simulink model "PassengerCar"  (R2019b)
settings: Solver=ode1  StartTime=0  StopTime=25  FixedStep=1.0000000000000000e-003  RelTol=1e-3
InitFcn:
  | sampleTime = str2double(get_param(bdroot, 'FixedStep'));
undefined symbols (not defined in the file or in its folder): AccPedalPos, BrakePedalPos, BrakeSwitch, DiscIntNeverNeededParam, DYNA4, EngSpd, IgnitionSwitch, InitialGear, InitialSpeed, IntendedEngTrq, LeftIndicator, MainBrakePress, MaxGear, MDL, MinGear, RefAcc, RefLane, RefLatPos, RefPath, RefPathCurv, RefSpd, RefSpdPreview, RefSpdRetrospect, RightIndicator, SteeringWheelAng, SteeringWheelTrq, UserDefinedRefValue, vm_const
libraries: UtilitiesLibrary x31, simulink x18, WheelSystemModules x13, LongitudinalControllerModules x13, LateralControllerModules x7, AnimationBusselectorModules x5, EnvironmentModules x5, BasicEngineControlModules x5, MiscellaneousControlModules x5, Animation3Modules x4, AuxiliariesModules x4, TireModules x4
(part 2 of 39)

== system PassengerCar/Animation ==
  fromCTRL : Inport
  fromControlUnits : Inport  Port=2
  fromTrailer : Inport  Port=3
  fromVehicle : Inport  Port=4
  fromTraffic : Inport  Port=5
  Animation3 : Animation3Modules/Animation3  DATA_NODE=MDL.Animation.Animation3
  AnimationContent : Animation3Modules/AnimationContentGeneric  SystemSampleTime=-1  Latency=0  AutoFrameSizeCalculation=off
  Bus Creator : BusCreator  Inputs=4
  DynaComponentInfo : Subsystem  Tag=DynaComponentInfo
      mask init:
      | data= get_param(gcb, 'UserData');
      settings: OpenFcn=DYNA4.ModelHandling.Component.ShowEditComponentInformationDialog(gcb);
      mask Display: disp(['Type = ', data.type, '\nGroup = ', data.group, '\nName = ', data.name ])
  Gauge Signals : AnimationBusselectorModules/Gauge Signals  SystemSampleTime=-1  Latency=0  AutoFrameSizeCalculation=off
  Open AnimationBusselectorModules : AnimationBusselectorModules/Open AnimationBusselectorModules  SystemSampleTime=-1  Latency=0  AutoFrameSizeCalculation=off
  Scenario Design : AnimationBusselectorModules/Scenario Design  SystemSampleTime=-1  Latency=0  AutoFrameSizeCalculation=off
  Terminator : Terminator
  Terminator1 : Terminator
  Terminator2 : Terminator
  Vehicle Light Signals : AnimationBusselectorModules/Vehicle Light Signals  SystemSampleTime=-1  VariantControl=AnimationData_Lights  Latency=0  AutoFrameSizeCalculation=off
  Vehicle Signals With Axles Animation : AnimationBusselectorModules/Vehicle Signals With Axles Animation  SystemSampleTime=-1  Latency=0  AutoFrameSizeCalculation=off
      settings: AttributesFormatString=requires veDYNA Chassis Component signals!
  wires:
  fromVehicle/1 -> Scenario Design/1, Vehicle Signals With Axles Animation/1, Gauge Signals/1
  fromCTRL/1 -> Scenario Design/2, Vehicle Light Signals/1
  fromTrailer/1 -> Terminator1/1
  fromControlUnits/1 -> Terminator2/1
  Vehicle Light Signals/1 -> Bus Creator/3
  Vehicle Signals With Axles Animation/1 -> Bus Creator/2
  Gauge Signals/1 -> Bus Creator/1
  Bus Creator/1 -> Animation3/1
  fromTraffic/1 -> Terminator/1
  Scenario Design/1 -> Bus Creator/4

== system PassengerCar/ComponentsOutput ==
  ControlUnits___UNIQUE_1 : Inport  Description=|
      | <name>ControlUnits</name>
      | <comment></comment>
  Trailer___UNIQUE_1 : Inport  Description=|  Port=2
      | <name>Trailer</name>
      | <comment></comment>
  Vehicle___UNIQUE_1 : Inport  Description=|  Port=3
      | <name>Vehicle</name>
      | <comment></comment>
  Environment___UNIQUE_1 : Inport  Description=|  Port=4
      | <name>Environment</name>
      | <comment></comment>
  Traffic___UNIQUE_1 : Inport  Description=|  Port=5
      | <name>Traffic</name>
      | <comment></comment>
  VehicleControl___UNIQUE_1 : Inport  Description=|  Port=6
      | <name>VehicleControl</name>
      | <comment></comment>
  __SRC__Components.(none) : Constant  Value=0.0  OutDataTypeStr=Inherit: Inherit via back propagation
  __TDO__Components : BusCreator  Inputs=7
  Components___UNIQUE_1 : Outport  Tag=TESIS DYNAware Component Bus Root  Description=|  VectorParamsAs1DForOutWhenUnconnected=off
      | <name></name>
      | <comment></comment>
  wires:
  __SRC__Components.(none)/1 -> __TDO__Components/1  "(none)"
  ControlUnits___UNIQUE_1/1 -> __TDO__Components/2  "ControlUnits"
  Trailer___UNIQUE_1/1 -> __TDO__Components/3  "Trailer"
  Vehicle___UNIQUE_1/1 -> __TDO__Components/4  "Vehicle"
  Environment___UNIQUE_1/1 -> __TDO__Components/5  "Environment"
  Traffic___UNIQUE_1/1 -> __TDO__Components/6  "Traffic"
  VehicleControl___UNIQUE_1/1 -> __TDO__Components/7  "VehicleControl"
  __TDO__Components/1 -> Components___UNIQUE_1/1  "Components"

== system PassengerCar/ControlUnits ==
  note: This component contains central control units that usually use bus communication
      | in the real vehicle to communicate with their physical counterpart.
      | Control units that are directly connected to their hardware counterpart such as
      | BrakeSystemControlUnit are located next to the corresponding physical component.
  fromCTRL : Inport
  fromTrailer : Inport  Port=2
  fromVehicle : Inport  Port=3
  fromTraffic : Inport  Port=4
  ADAS : Subsystem
  ControlUnitsOutput : Subsystem  Tag=TESIS DYNAware Interface Block  mask{NeedsUpdate=off, SignalInfo=|}
      mask SignalInfo=|
      | {
      |   "Version": "4.6",
      |   "MuxedOutputBusName": "ControlUnits",
      |   "MuxedInputBusName": "input",
      |   "MuxedInputSelected": false,
      |   "MuxedOutputSelected": true,
      |   "SignalData": [
      |     {
      |       "initialValue": "0.0",
      |       "name": "VCU",
      |       "comment": "",
      |       "minString": "",
      |       "maxString": "",
      |       "width": -1,
      |       "dataType": 0,
      |       "signalType": 1,
      |       "createSignal": false,
      |       "outputName": "VCU",
      |       "generateSignalAccessBlock": false,
      |       "accessId": "$(parentId).$(blockName).$(outputName)"
      |     },
      |     {
      |       "initialValue": "0.0",
      |       "name": "ADAS",
      |       "comment": "",
      |       "minString": "",
      |       "maxString": "",
      |       "width": -1,
      |       "dataType": 0,
      |       "signalType": 1,
      |       "createSignal": false,
      |       "outputName": "ADAS",
      |       "generateSignalAccessBlock": false,
      |       "accessId": "$(parentId).$(blockName).$(outputName)"
      |     },
      |     {
      |       "initialValue": "0.0",
      |       "name": "LCU",
      |       "comment": "",
      |       "minString": "",
      |       "maxString": "",
      |       "width": -1,
      |       "dataType": 0,
      |       "signalType": 1,
      |       "createSignal": false,
      |       "outputName": "LCU",
      |       "generateSignalAccessBlock": false,
      |       "accessId": "$(parentId).$(blockName).$(outputName)"
      |     },
      |     {
      |       "initialValue": "0.0",
      |       "name": "StateSensors",
      |       "comment": "",
      |       "minString": "",
      |       "maxString": "",
      |       "width": -1,
      |       "dataType": 0,
      |       "signalType": 1,
      |       "createSignal": false,
      |       "outputName": "StateSensors",
      |       "generateSignalAccessBlock": false,
      |       "accessId": "$(parentId).$(blockName).$(outputName)"
      |     }
      |   ]
      | }
      mask prompts: NeedsUpdate "Specify, if subsystem content needs to be updated"; SignalInfo "Signal Info (json)"
      mask help: DYNA4 Interface Block Version 4.6
      mask init:
      | blockName = get_param(gcbh, 'Name');
      | parentId = DYNA4.ModelHandling.AccessID.getFromHierarchy(gcbh);
      | TD.InterfaceBlock.ModelCallbacks.GenerateContent(gcb);
      settings: DeleteFcn=TD.InterfaceBlock.ModelCallbacks.CloseGUI( gcbh );  NameChangeFcn=TD.InterfaceBlock.ModelCallbacks.BlockRenamedHandler(gcbh);  OpenFcn=TD.InterfaceBlock.ModelCallbacks.OpenGUI( gcbh );  CloseFcn=TD.InterfaceBlock.ModelCallbacks.CloseGUI( gcbh );
      mask Display:
      | image('InterfaceBlock.png','center');
      | port_label('input',1, 'VCU');
      | port_label('input',2, 'ADAS');
      | port_label('input',3, 'LCU');
      | port_label('input',4, 'StateSensors');
      | port_label('output',1, 'ControlUnits');
  DynaComponentInfo : Subsystem  Tag=DynaComponentInfo
      mask init:
      | data= get_param(gcb, 'UserData');
      settings: OpenFcn=DYNA4.ModelHandling.Component.ShowEditComponentInformationDialog(gcb);
      mask Display: disp(['Type = ', data.type, '\nGroup = ', data.group, '\nName = ', data.name ])
  LCU : Subsystem
  StateSensors : Subsystem
  TraceMarker : UtilitiesLibrary/DYNA4 Trace Marker  Tag=DYNA4_TRACE_MARKER  SettingType=Standard  PrefixModelBlockID=on  PrefixRootSignalName=off  NamePattern='$(modelBlockID).$(rootSignalName)'
  VCU : Subsystem
  ControlUnits : Outport  VectorParamsAs1DForOutWhenUnconnected=off
  wires:
  fromTraffic/1 -> StateSensors/4(fromTraffic)
  fromTrailer/1 -> StateSensors/2(fromTrailer)
  fromVehicle/1 -> ADAS/2(fromVehicle), LCU/2(fromVehicle), StateSensors/3(fromVehicle), VCU/2(fromVehicle)
  fromCTRL/1 -> ADAS/1(fromCTRL), LCU/1(fromCTRL), StateSensors/1(fromCTRL), VCU/1(fromCTRL)
  LCU/1(LCU) -> ControlUnitsOutput/3(LCU___UNIQUE_1)
  ControlUnitsOutput/1(ControlUnits___UNIQUE_1) -> ControlUnits/1, TraceMarker/1
  ADAS/1(ADAS) -> ControlUnitsOutput/2(ADAS___UNIQUE_1), VCU/3(fromADAS)
  VCU/1(VCU) -> ControlUnitsOutput/1(VCU___UNIQUE_1)
  StateSensors/1(StateSensors) -> ControlUnitsOutput/4(StateSensors___UNIQUE_1)

== system PassengerCar/DYNA4 Logo ==

== system PassengerCar/Environment ==
  fromCTRL : Inport
  fromTrailer : Inport  Port=2
  fromVehicle : Inport  Port=3
  fromTraffic : Inport  Port=4
  AdditionalRoadElevation : EnvironmentModules/AdditionalRoadElevation  DATA_NODE=MDL.Environment.AdditionalRoadElevation  AddLongRoadSlope=MDL.Environment.AdditionalRoadElevation.AddLongRoadSlope  AddLatRoadSlope=MDL.Environment.AdditionalRoadElevation.AddLatRoadSlope  FrontLeftAddRoadElev=MDL.Environment.AdditionalRoadElevation.FrontLeftAddRoadElev  FrontRightAddRoadElev=MDL.Environment.AdditionalRoadElevation.FrontRightAddRoadElev  RearLeftAddRoadElev=MDL.Environment.AdditionalRoadElevation.RearLeftAddRoadElev  RearRightAddRoadElev=MDL.Environment.AdditionalRoadElevation.RearRightAddRoadElev  Rear2LeftAddRoadElev=MDL.Environment.AdditionalRoadElevation.Rear2LeftAddRoadElev  Rear2RightAddRoadElev=MDL.Environment.AdditionalRoadElevation.Rear2RightAddRoadElev  Rear3LeftAddRoadElev=MDL.Environment.AdditionalRoadElevation.Rear3LeftAddRoadElev  Rear3RightAddRoadElev=MDL.Environment.AdditionalRoadElevation.Rear3RightAddRoadElev  TrailerFrontLeftAddRoadElev=MDL.Environment.AdditionalRoadElevation.TrailerFrontLeftAddRoadElev  TrailerFrontRightAddRoadElev=MDL.Environment.AdditionalRoadElevation.TrailerFrontRightAddRoadElev  TrailerRearLeftAddRoadElev=MDL.Environment.AdditionalRoadElevation.TrailerRearLeftAddRoadElev  TrailerRearRightAddRoadElev=MDL.Environment.AdditionalRoadElevation.TrailerRearRightAddRoadElev  TrailerRear2LeftAddRoadElev=MDL.Environment.AdditionalRoadElevation.TrailerRear2LeftAddRoadElev  TrailerRear2RightAddRoadElev=MDL.Environment.AdditionalRoadElevation.TrailerRear2RightAddRoadElev  TrailerRear3LeftAddRoadElev=MDL.Environment.AdditionalRoadElevation.TrailerRear3LeftAddRoadElev  TrailerRear3RightAddRoadElev=MDL.Environment.AdditionalRoadElevation.TrailerRear3RightAddRoadElev  AbscissaTypes=MDL.Environment.AdditionalRoadElevation.AbscissaTypes  SelectDistanceAbscissaType=MDL.Environment.AdditionalRoadElevation.SelectDistanceAbscissaType  IsActive=MDL.Environment.AdditionalRoadElevation.IsActive
  AmbientConditions : EnvironmentModules/AmbientConditions  DATA_NODE=MDL.Environment.AmbientConditions  Temp=MDL.Environment.AmbientConditions.Temp  RefPress=MDL.Environment.AmbientConditions.Pressure.RefPress  AmbPress=MDL.Environment.AmbientConditions.Pressure.AmbPress  RelAirHumidity=MDL.Environment.AmbientConditions.RelAirHumidity
  AnimationContent : Animation3Modules/AnimationContentEnvironment  SystemSampleTime=-1  Latency=0  AutoFrameSizeCalculation=off
  DynaComponentInfo : Subsystem  Tag=DynaComponentInfo
      mask init:
      | data= get_param(gcb, 'UserData');
      settings: OpenFcn=DYNA4.ModelHandling.Component.ShowEditComponentInformationDialog(gcb);
      mask Display: disp(['Type = ', data.type, '\nGroup = ', data.group, '\nName = ', data.name ])
  EnvironmentInputs : EnvironmentModules/EnvironmentInputs  SystemSampleTime=-1  Latency=0  AutoFrameSizeCalculation=off
  EnvironmentOutput : Subsystem  Tag=TESIS DYNAware Interface Block  mask{NeedsUpdate=off, SignalInfo=|}
      mask SignalInfo=|
      | {
      |   "Version": "4.6",
      |   "MuxedOutputBusName": "Environment",
      |   "MuxedInputBusName": "input",
      |   "MuxedInputSelected": false,
      |   "MuxedOutputSelected": true,
      |   "SignalData": [
      |     {
      |       "initialValue": "0.0",
      |       "name": "WindImpact",
      |       "comment": "",
      |       "minString": "",
      |       "maxString": "",
      |       "width": -1,
      |       "dataType": 0,
      |       "signalType": 1,
      |       "createSignal": false,
      |       "outputName": "WindImpact",
      |       "generateSignalAccessBlock": false,
      |       "accessId": "$(parentId).$(blockName).$(outputName)"
      |     },
      |     {
      |       "initialValue": "0.0",
      |       "name": "RoadFrictionScaling",
      |       "comment": "",
      |       "minString": "",
      |       "maxString": "",
      |       "width": -1,
      |       "dataType": 0,
      |       "signalType": 1,
      |       "createSignal": false,
      |       "outputName": "RoadFrictionScaling",
      |       "generateSignalAccessBlock": false,
      |       "accessId": "$(parentId).$(blockName).$(outputName)"
      |     },
      |     {
      |       "initialValue": "0.0",
      |       "name": "AdditionalRoadElevation",
      |       "comment": "",
      |       "minString": "",
      |       "maxString": "",
      |       "width": -1,
      |       "dataType": 0,
      |       "signalType": 1,
      |       "createSignal": false,
      |       "outputName": "AdditionalRoadElevation",
      |       "generateSignalAccessBlock": false,
      |       "accessId": "$(parentId).$(blockName).$(outputName)"
      |     },
      |     {
      |       "initialValue": "0.0",
      |       "name": "AmbientConditions",
      |       "comment": "",
      |       "minString": "",
      |       "maxString": "",
      |       "width": -1,
      |       "dataType": 0,
      |       "signalType": 1,
      |       "createSignal": false,
      |       "outputName": "AmbientConditions",
      |       "generateSignalAccessBlock": false,
      |       "accessId": "$(parentId).$(blockName).$(outputName)"
      |     }
      |   ]
      | }
      mask prompts: NeedsUpdate "Specify, if subsystem content needs to be updated"; SignalInfo "Signal Info (json)"
      mask help: DYNA4 Interface Block Version 4.6
      mask init:
      | blockName = get_param(gcbh, 'Name');
      | parentId = DYNA4.ModelHandling.AccessID.getFromHierarchy(gcbh);
      | TD.InterfaceBlock.ModelCallbacks.GenerateContent(gcb);
      settings: DeleteFcn=TD.InterfaceBlock.ModelCallbacks.CloseGUI( gcbh );  NameChangeFcn=TD.InterfaceBlock.ModelCallbacks.BlockRenamedHandler(gcbh);  OpenFcn=TD.InterfaceBlock.ModelCallbacks.OpenGUI( gcbh );  CloseFcn=TD.InterfaceBlock.ModelCallbacks.CloseGUI( gcbh );
      mask Display:
      | image('InterfaceBlock.png','center');
      | port_label('input',1, 'WindImpact');
      | port_label('input',2, 'RoadFrictionScaling');
      | port_label('input',3, 'AdditionalRoadElevation');
      | port_label('input',4, 'AmbientConditions');
      | port_label('output',1, 'Environment');
  Road : Subsystem
  RoadFrictionScaling : EnvironmentModules/RoadFrictionScaling  DATA_NODE=MDL.Environment.RoadFrictionScaling  SimulationTerminationSwitch=MDL.Environment.RoadFrictionScaling.Scheduler.SimulationTerminationSwitch  Phase=MDL.Environment.RoadFrictionScaling.Scheduler.Phase
  TraceMarker : UtilitiesLibrary/DYNA4 Trace Marker  Tag=DYNA4_TRACE_MARKER  SettingType=Standard  PrefixModelBlockID=on  PrefixRootSignalName=off  NamePattern='$(modelBlockID).$(rootSignalName)'
  WindImpact : EnvironmentModules/WindImpact  DATA_NODE=MDL.Environment.WindImpact  SimulationTerminationSwitch=MDL.Environment.WindImpact.Scheduler.SimulationTerminationSwitch  Phase=MDL.Environment.WindImpact.Scheduler.Phase
  Environment : Outport  VectorParamsAs1DForOutWhenUnconnected=off
  wires:
  EnvironmentInputs/10 -> AdditionalRoadElevation/8
  EnvironmentInputs/9 -> AdditionalRoadElevation/7
  fromTrailer/1 -> EnvironmentInputs/2
  fromVehicle/1 -> EnvironmentInputs/1
  AdditionalRoadElevation/1 -> EnvironmentOutput/3(AdditionalRoadElevation___UNIQUE_1)
  EnvironmentInputs/1 -> WindImpact/1, RoadFrictionScaling/1
  EnvironmentInputs/2 -> WindImpact/2, RoadFrictionScaling/2
  WindImpact/1 -> EnvironmentOutput/1(WindImpact___UNIQUE_1)
  RoadFrictionScaling/1 -> EnvironmentOutput/2(RoadFrictionScaling___UNIQUE_1)
  EnvironmentOutput/1(Environment___UNIQUE_1) -> Environment/1, TraceMarker/1
  EnvironmentInputs/4 -> AdditionalRoadElevation/2
  fromCTRL/1 -> EnvironmentInputs/4
  EnvironmentInputs/7 -> AdditionalRoadElevation/5
  EnvironmentInputs/8 -> AdditionalRoadElevation/6
  EnvironmentInputs/5 -> AdditionalRoadElevation/3
  EnvironmentInputs/6 -> AdditionalRoadElevation/4
  fromTraffic/1 -> EnvironmentInputs/3
  EnvironmentInputs/3 -> AmbientConditions/1, AdditionalRoadElevation/1
  EnvironmentInputs/11 -> AmbientConditions/2
  AmbientConditions/1 -> EnvironmentOutput/4(AmbientConditions___UNIQUE_1)

== system PassengerCar/SimulationControl ==
  note: DYNA4 Simulation Control
  note: COPYRIGHT by Vector Informatik GmbH
  DYNA4 Simulation Control : SimulationControlLibrary/DYNA4 Simulation Control  Tag=vedynaSimctrlMask  sampleTime=sampleTime  stopTime=MDL.SimulationControl.StopTime.v  traceInterval=MDL.SimulationControl.TraceInterval.v  consoleOutputDownsampling=MDL.SimulationControl.ConsoleOutputDownsampling.v  realTimeFactor=-1
  DynaComponentInfo : Subsystem  Tag=DynaComponentInfo
      mask init:
      | data= get_param(gcb, 'UserData');
      settings: OpenFcn=DYNA4.ModelHandling.Component.ShowEditComponentInformationDialog(gcb);
      mask Display: disp(['Type = ', data.type, '\nGroup = ', data.group, '\nName = ', data.name ])
